simulink model "mdl_6_1_1"  (R2022b)
settings: Solver=VariableStepAuto  StartTime=0.0  StopTime=4  MaxStep=0.001  RelTol=1e-3
settings Model: Creator=jack  LastModifiedBy=jackyeh

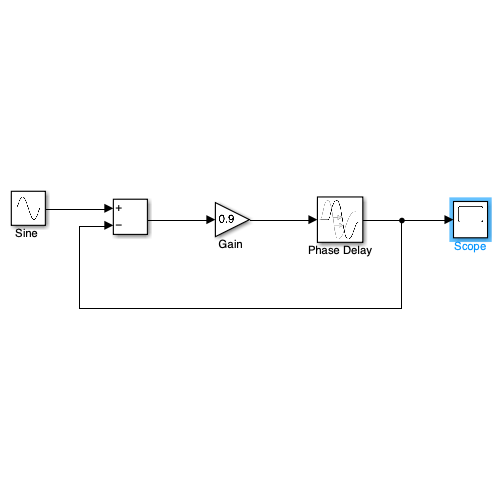
[thumbnail: Simulink's stored preview of the top-level diagram]
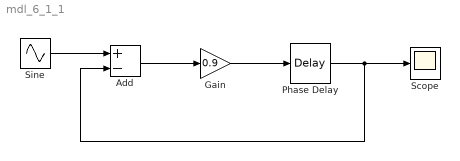
== system mdl_6_1_1 ==
  Add : Sum  Inputs=+-
  "Gain " : Gain  Gain=0.9
  Phase Delay : TransportDelay  DelayTime=(1/50)*0.5
  Scope : Scope
  "Sine " : Sin  Frequency=2*pi*50  SampleTime=0
  wires:
  "Sine "/1 -> Add/1
  Add/1 -> "Gain "/1
  "Gain "/1 -> Phase Delay/1
  Phase Delay/1 -> Scope/1, Add/2
